simulink model "BolandLab2"  (R2024a)
settings: Solver=VariableStepAuto  StartTime=0.0  StopTime=100  RelTol=1e-3
settings Model: Creator=Test  LastModifiedBy=Test

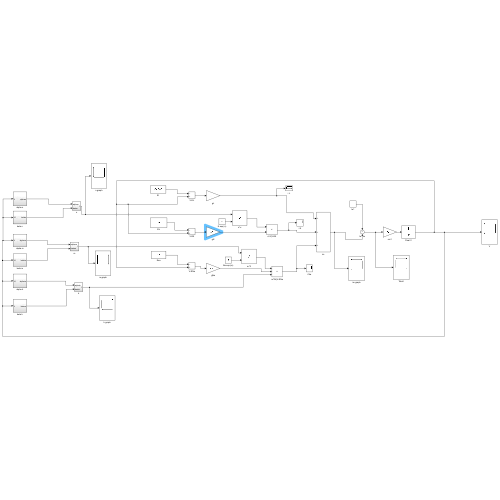
[thumbnail: Simulink's stored preview of the top-level diagram]
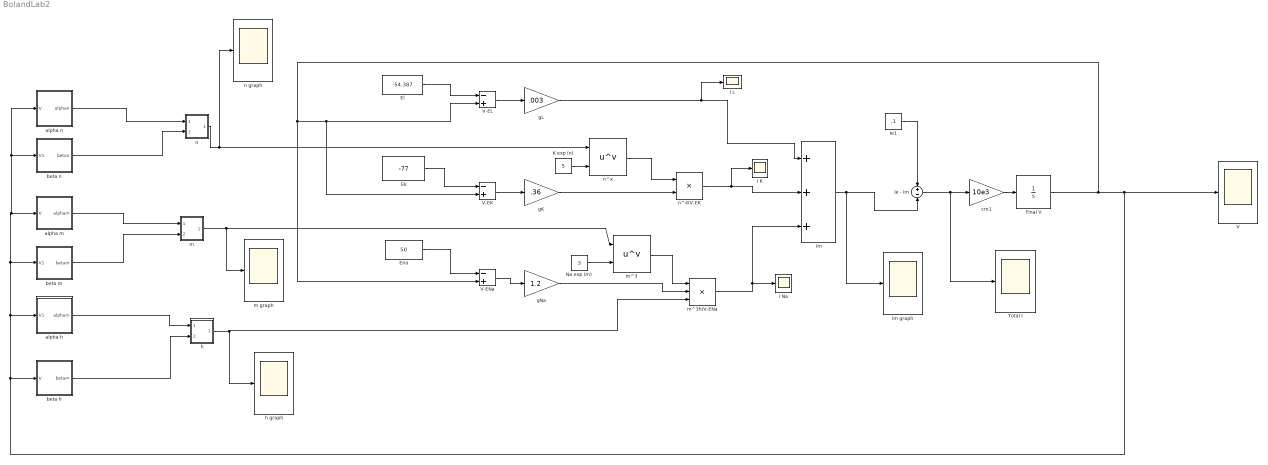
== system BolandLab2 ==
  Ek : Constant  Value=-77
  "El " : Constant  Value=-54.387
  "Ena " : Constant  Value=50
  Final V : Integrator  InitialCondition=-54.387
  Ie - im : Sum  Inputs=+-
  Ie1 : Constant  Value=.1
  K exp (n) : Constant  Value=5
  Na exp (m) : Constant  Value=3
  Total I : Scope
  V : Scope
  V-EK : Sum  Inputs=-+
  V-EL : Sum  Inputs=-+
  V-ENa : Sum  Inputs=-+
  alpha h : Subsystem
  alpha m : Subsystem
  alpha n : Subsystem
  beta h : Subsystem
  beta m : Subsystem
  beta n : Subsystem
  cm1 : Gain  Gain=10e3
  gK : Gain  Gain=.36
  gL : Gain  Gain=.003
  gNa : Gain  Gain=1.2
  h : Subsystem
  h graph : Scope
  i K : Scope
  i L : Scope
  i Na : Scope
  im : Sum  Inputs=+++
  im graph : Scope
  m : Subsystem
  m graph : Scope
  m^3 : Math  Operator=pow
  m^3h(V-ENa : Product  Inputs=3
  n : Subsystem
  n graph : Scope
  n^4(V-EK : Product
  n^x : Math  Operator=pow
  wires:
  alpha n/1(alphan) -> n/1(alphan)
  beta n/1(betan) -> n/2(betan)
  alpha m/1(alpham) -> m/1(alpham)
  beta m/1(betam) -> m/2(betam)
  beta h/1(betam) -> h/2(betah)
  alpha h/1(alpham) -> h/1(alphah)
  "El "/1 -> V-EL/1
  Ek/1 -> V-EK/1
  "Ena "/1 -> V-ENa/1
  V-EL/1 -> gL/1
  V-EK/1 -> gK/1
  V-ENa/1 -> gNa/1
  n/1(Out1) -> n graph/1, n^x/1
  K exp (n)/1 -> n^x/2
  n^x/1 -> n^4(V-EK/1
  gK/1 -> n^4(V-EK/2
  gL/1 -> i L/1, im/1
  n^4(V-EK/1 -> i K/1, im/2
  m/1(Out1) -> m graph/1, m^3/1
  Na exp (m)/1 -> m^3/2
  m^3h(V-ENa/1 -> i Na/1, im/3
  m^3/1 -> m^3h(V-ENa/1
  gNa/1 -> m^3h(V-ENa/2
  h/1(Out1) -> h graph/1, m^3h(V-ENa/3
  im/1 -> im graph/1, Ie - im/2
  Ie1/1 -> Ie - im/1
  Ie - im/1 -> Total I/1, cm1/1
  Final V/1 -> V/1, alpha n/1(V), beta n/1(V1), alpha m/1(V), beta m/1(V1), alpha h/1(V1), beta h/1(V), V-ENa/2, V-EK/2, V-EL/2
  cm1/1 -> Final V/1

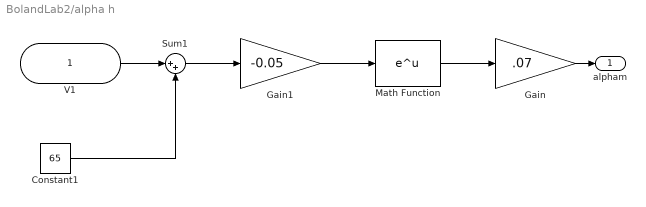
== system BolandLab2/alpha h ==
  V1 : Inport
  Constant1 : Constant  Value=65
  Gain : Gain  Gain=.07
  Gain1 : Gain  Gain=-0.05
  Math Function : Math
  Sum1 : Sum  Inputs=|++
  alpham : Outport
  wires:
  Constant1/1 -> Sum1/2
  V1/1 -> Sum1/1
  Math Function/1 -> Gain/1
  Gain1/1 -> Math Function/1
  Gain/1 -> alpham/1
  Sum1/1 -> Gain1/1

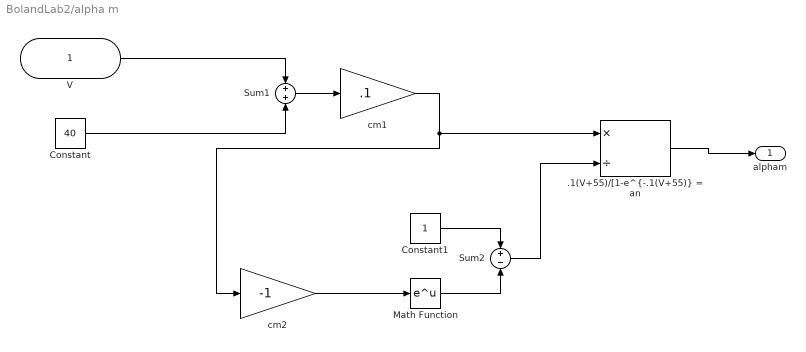
== system BolandLab2/alpha m ==
  V : Inport
  ".1(V+55)/[1-e^{-.1(V+55)} = an" : Product  Inputs=*/
  Constant : Constant  Value=40
  Constant1 : Constant
  Math Function : Math
  Sum1 : Sum
  Sum2 : Sum  Inputs=+-
  cm1 : Gain  Gain=.1
  cm2 : Gain  Gain=-1
  alpham : Outport
  wires:
  Sum2/1 -> ".1(V+55)/[1-e^{-.1(V+55)} = an"/2
  cm2/1 -> Math Function/1
  cm1/1 -> ".1(V+55)/[1-e^{-.1(V+55)} = an"/1, cm2/1
  Math Function/1 -> Sum2/2
  Sum1/1 -> cm1/1
  Constant1/1 -> Sum2/1
  Constant/1 -> Sum1/2
  V/1 -> Sum1/1
  ".1(V+55)/[1-e^{-.1(V+55)} = an"/1 -> alpham/1

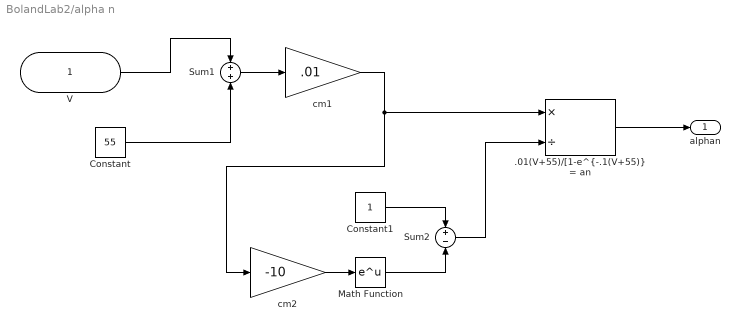
== system BolandLab2/alpha n ==
  V : Inport
  ".01(V+55)/[1-e^{-.1(V+55)} = an" : Product  Inputs=*/
  Constant : Constant  Value=55
  Constant1 : Constant
  Math Function : Math
  Sum1 : Sum
  Sum2 : Sum  Inputs=+-
  cm1 : Gain  Gain=.01
  cm2 : Gain  Gain=-10
  alphan : Outport
  wires:
  Sum2/1 -> ".01(V+55)/[1-e^{-.1(V+55)} = an"/2
  cm2/1 -> Math Function/1
  cm1/1 -> ".01(V+55)/[1-e^{-.1(V+55)} = an"/1, cm2/1
  Math Function/1 -> Sum2/2
  Sum1/1 -> cm1/1
  Constant1/1 -> Sum2/1
  Constant/1 -> Sum1/2
  V/1 -> Sum1/1
  ".01(V+55)/[1-e^{-.1(V+55)} = an"/1 -> alphan/1

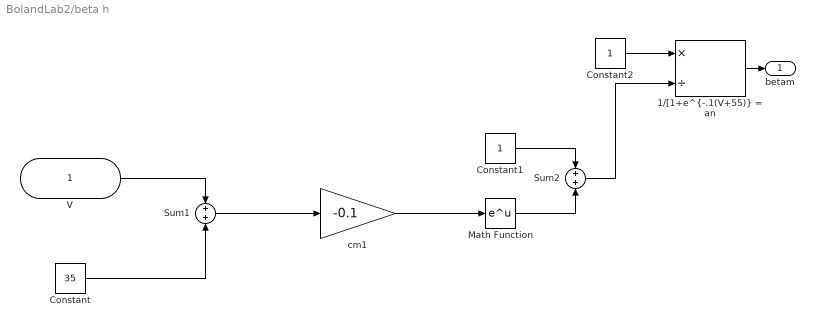
== system BolandLab2/beta h ==
  V : Inport
  "1/[1+e^{-.1(V+55)} = an" : Product  Inputs=*/
  Constant : Constant  Value=35
  Constant1 : Constant
  Constant2 : Constant
  Math Function : Math
  Sum1 : Sum
  Sum2 : Sum
  cm1 : Gain  Gain=-0.1
  betam : Outport
  wires:
  Sum2/1 -> "1/[1+e^{-.1(V+55)} = an"/2
  cm1/1 -> Math Function/1
  Math Function/1 -> Sum2/2
  Sum1/1 -> cm1/1
  Constant1/1 -> Sum2/1
  Constant/1 -> Sum1/2
  V/1 -> Sum1/1
  "1/[1+e^{-.1(V+55)} = an"/1 -> betam/1
  Constant2/1 -> "1/[1+e^{-.1(V+55)} = an"/1

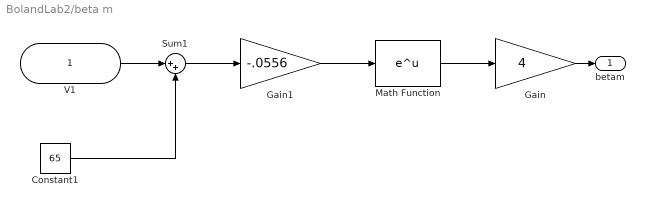
== system BolandLab2/beta m ==
  V1 : Inport
  Constant1 : Constant  Value=65
  Gain : Gain  Gain=4
  Gain1 : Gain  Gain=-.0556
  Math Function : Math
  Sum1 : Sum  Inputs=|++
  betam : Outport
  wires:
  Constant1/1 -> Sum1/2
  V1/1 -> Sum1/1
  Math Function/1 -> Gain/1
  Gain1/1 -> Math Function/1
  Gain/1 -> betam/1
  Sum1/1 -> Gain1/1

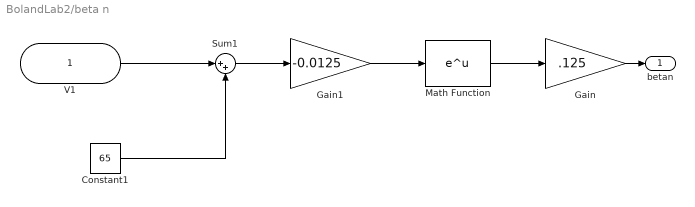
== system BolandLab2/beta n ==
  V1 : Inport
  Constant1 : Constant  Value=65
  Gain : Gain  Gain=.125
  Gain1 : Gain  Gain=-0.0125
  Math Function : Math
  Sum1 : Sum  Inputs=|++
  betan : Outport
  wires:
  Constant1/1 -> Sum1/2
  V1/1 -> Sum1/1
  Math Function/1 -> Gain/1
  Gain1/1 -> Math Function/1
  Gain/1 -> betan/1
  Sum1/1 -> Gain1/1

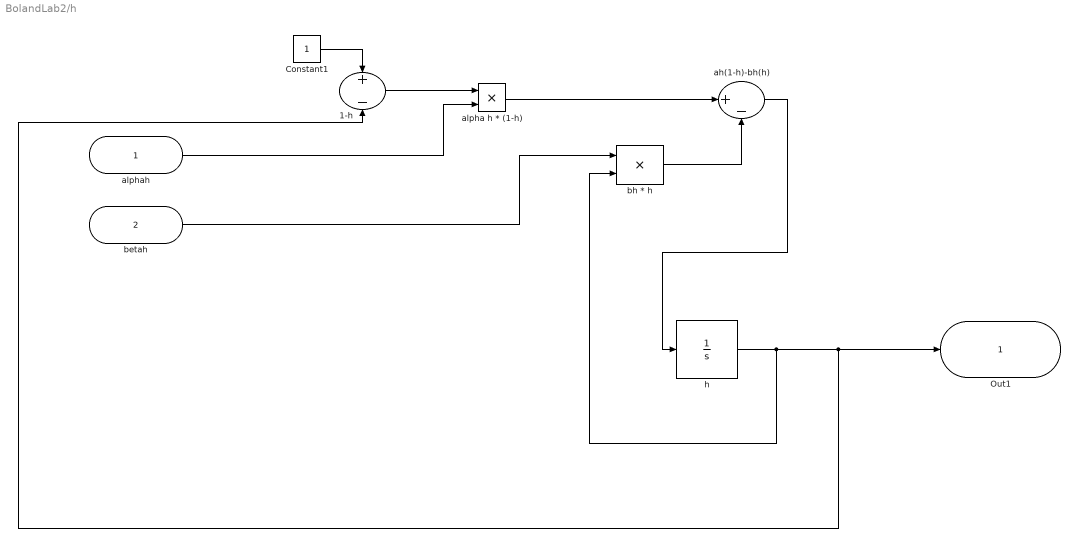
== system BolandLab2/h ==
  alphah : Inport
  betah : Inport  Port=2
  1-h : Sum  Inputs=+-
  Constant1 : Constant
  ah(1-h)-bh(h) : Sum  Inputs=|+-
  alpha h * (1-h) : Product
  bh * h : Product
  h : Integrator  InitialCondition=.1
  Out1 : Outport
  wires:
  ah(1-h)-bh(h)/1 -> h/1
  betah/1 -> bh * h/1
  alphah/1 -> alpha h * (1-h)/2
  1-h/1 -> alpha h * (1-h)/1
  alpha h * (1-h)/1 -> ah(1-h)-bh(h)/1
  Constant1/1 -> 1-h/1
  bh * h/1 -> ah(1-h)-bh(h)/2
  h/1 -> bh * h/2, Out1/1, 1-h/2

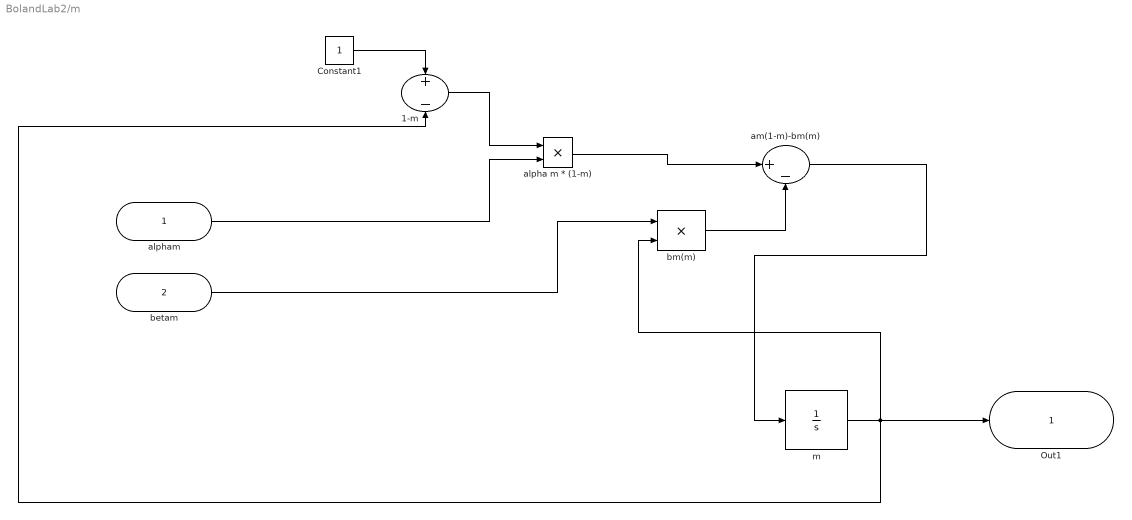
== system BolandLab2/m ==
  alpham : Inport
  betam : Inport  Port=2
  1-m : Sum  Inputs=+-
  Constant1 : Constant
  alpha m * (1-m) : Product
  am(1-m)-bm(m) : Sum  Inputs=|+-
  bm(m) : Product
  m : Integrator  InitialCondition=.3
  Out1 : Outport
  wires:
  am(1-m)-bm(m)/1 -> m/1
  betam/1 -> bm(m)/1
  alpham/1 -> alpha m * (1-m)/2
  1-m/1 -> alpha m * (1-m)/1
  m/1 -> Out1/1, bm(m)/2, 1-m/2
  alpha m * (1-m)/1 -> am(1-m)-bm(m)/1
  Constant1/1 -> 1-m/1
  bm(m)/1 -> am(1-m)-bm(m)/2

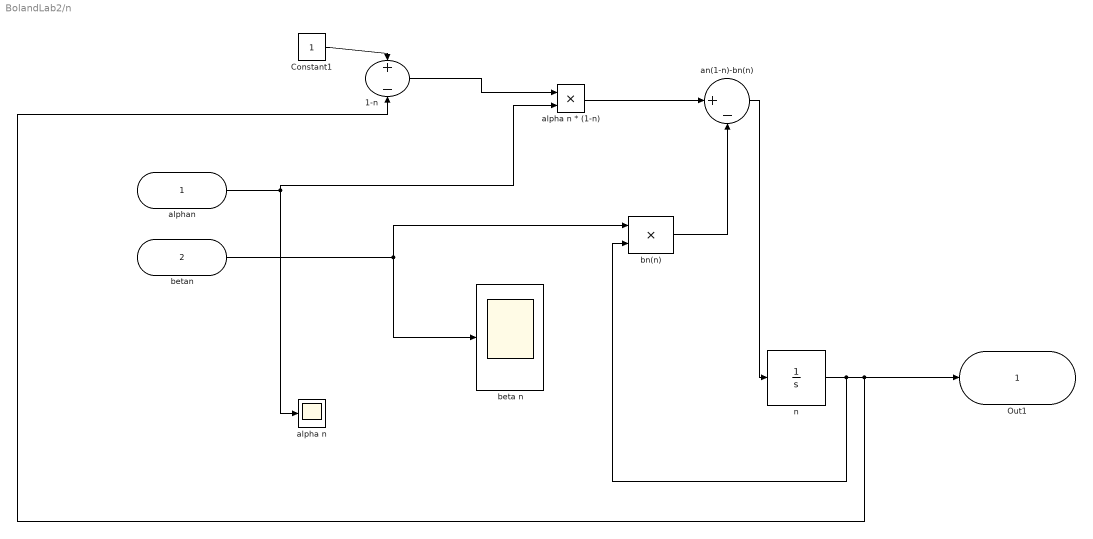
== system BolandLab2/n ==
  alphan : Inport
  betan : Inport  Port=2
  1-n : Sum  Inputs=+-
  Constant1 : Constant
  alpha n : Scope
  alpha n * (1-n) : Product
  an(1-n)-bn(n) : Sum  Inputs=|+-
  beta n : Scope
  bn(n) : Product
  n : Integrator  InitialCondition=.45
  Out1 : Outport
  wires:
  an(1-n)-bn(n)/1 -> n/1
  betan/1 -> beta n/1, bn(n)/1
  alphan/1 -> alpha n/1, alpha n * (1-n)/2
  1-n/1 -> alpha n * (1-n)/1
  alpha n * (1-n)/1 -> an(1-n)-bn(n)/1
  Constant1/1 -> 1-n/1
  bn(n)/1 -> an(1-n)-bn(n)/2
  n/1 -> 1-n/2, Out1/1, bn(n)/2
